simulink model "IEEE34bus_v2019b_Discrete_ZIPload"  (R2019b)
settings: Solver=ode4  StartTime=0.0  StopTime=5  FixedStep=Ts  MaxStep=1e-4  RelTol=1e-4
InitFcn:
  | a=1; % Loading Factor
  | Ts=50e-6;
  | % phase to sequence conversion of RXB matrices
  | c=1*exp(sqrt(-1)*(120*pi/180));
  | T=[1 1 1;1 c*c c;1 c c*c];
  | Tinv=1/3*[1 1 1;1 c c*c;1 c*c c];
  | 
  | % Simulation data for the IEEE 34 Node Test Feeder model
  | mi2km = 1.60934;%  miles to km conversion
  | ft2km = 0.0003048; % feet to km conversion
  | ms2F = 1*1e-6/(2*pi*60);% microsiemens to Farads conversion
  | 
  | %% Configuration 300 - series reactance - ohm/mile
  | R_300 = [1.3368 0.2101 0.2130;0.2101 1.3238 0.2066;0.2130 0.2066 1.3294];
  | X_300 = [1.3343 0.5779 0.5015;0.5779 1.3569 0.4591;0.5015 0.4591 1.3471];
  | % charging susceptance - microsiemens/mile
  | B_300 = [5.3350 -1.5313 -0.9943;-1.5313 5.0979 -0.6212;-0.9943 -0.6212 4.8880];
  | 
  | R_300 = R_300/mi2km;
  | Rseq=Tinv*R_300*T;
  | R1_300=Rseq(2,2);R0_300=Rseq(1,1);
  | 
  | L_300 = (X_300/(2*pi*60))/mi2km;
  | Lseq=Tinv*L_300*T;
  | L1_300=Lseq(2,2);L0_300=Lseq(1,1);
  | 
  | C_300 =(B_300*ms2F)/mi2km;
  | Cseq=Tinv*C_300*T;
  | C1_300=Cseq(2,2);C0_300=Cseq(1,1);
  | 
  | %% Configuration 301 - series reactance - ohm/mile
  | R_301 = [1.9300 0.2327 0.2359;0.2327 1.9157 0.2288;0.2359 0.2288 1.9219];
  | X_301 = [1.4115 0.6442 0.5691;0.6442 1.4281 0.5238;0.5691 0.5238 1.4209];
  | % charging susceptance - microsiemens/mile
  | B_301 = [5.1207 -1.4364 -0.9402;-1.4364 4.9055 -0.5951;-0.9402 -0.5951 4.7154];
  | 
  | R_301 = R_301/mi2km;
  | Rseq=Tinv*R_301*T;
  | R1_301=Rseq(2,2);R0_301=Rseq(1,1);
  | 
  | L_301 = (X_301/(2*pi*60))/mi2km;
  | Lseq=Tinv*L_301*T;
  | L1_301=Lseq(2,2);L0_301=Lseq(1,1);
  | 
  | C_301 =(B_301*ms2F)/mi2km;
  | Cseq=Tinv*C_301*T;
  | C1_301=Cseq(2,2);C0_301=Cseq(1,1);
  | 
  | %% Configuration 302 - series reactance - ohm/mile
  | R_302 = [2.7995 0 0;0 0 0;0 0 0];
  | X_302 = [1.4855 0 0;0 0 0;0 0 0];
  | % charging susceptance - microsiemens/mile
  | B_302 = [4.2251 0 0;0 0 0;0 0 0];
  | 
  | R_302 = R_302/mi2km;
  | Rseq=Tinv*R_302*T;
  | R1_302=Rseq(2,2);R0_302=Rseq(1,1);
  | 
  | L_302 = (X_302/(2*pi*60))/mi2km;
  | Lseq=Tinv*L_302*T;
  | ... (+41 lines)
undefined symbols (not defined in the file): find_system
libraries: powerlib x552, powerlib_meascontrol x162
(part 9 of 9)

== matlab function IEEE34bus_v2019b_Discrete_ZIPload/860 D PQ/Embedded MATLAB Function1 ==
  data: Iinjinst output; Vmeas input; LoadType parameter; Vnom parameter; Pnom parameter; Qnom parameter; Vlim parameter; fnom parameter; clock input; Ddel input
%Three Phase Delta ZIP Load
%Author: Arun Suresh, University of North Carolina, Charlotte
%Pl=Pnom(Kz*(Vmeas/Vnom)^2+Ki(Vmeas/Vnom)+Kp), nom-nominal value,meas-measured value
%Ql=Qnom(Kz*(Vmeas/Vnom)^2+Ki(Vmeas/Vnom)+Kp), nom-nominal value,meas-measured value
%Iinj=((Pl+jQl)/Vmeas)'
function Iinjinst  = InjectedCurrent(Vmeas,LoadType,Vnom,Pnom,Qnom,Vlim,fnom,clock,Ddel)
% Calculate Pl and Ql.
Kz=0;Ki=0;Kp=0;
Vk=abs(Vmeas/(Vnom));%(Vmeas/Vnom)
switch LoadType  % 1 for Constant Z, 2 for Constant I and 3 for Constant P, 
    case 1
        Kz=1;
    case 2
        if Vk >= Vlim % convert to Constant Z load due to voltage violation
            Ki=1;
        else
            Kz=1;
        end
    case 3
        if Vk >= Vlim % convert to Constant Z load due to voltage violation
           Kp=1;
        else
            Kz=1;
        end          
 
end
Pl=Pnom'.*((Kz*Vk.*Vk)+(Ki*Vk)+(Kp));
Ql=Qnom'.*((Kz*Vk.*Vk)+(Ki*Vk)+(Kp));
% Net Injected Curent.
% j=sqrt(-1);
Iinj = conj((Pl+j*Ql)./Vmeas);
Iinjinsta =abs(Iinj(1))*sqrt(2)*sin(2*fnom*pi*clock + angle(Iinj(1))+Ddel(1));
Iinjinstb =abs(Iinj(2))*sqrt(2)*sin(2*fnom*pi*clock + angle(Iinj(2))+Ddel(2));
Iinjinstc =abs(Iinj(3))*sqrt(2)*sin(2*fnom*pi*clock + angle(Iinj(3))+Ddel(3));
Iinjinst=[Iinjinsta  Iinjinstb  Iinjinstc]';

== matlab function IEEE34bus_v2019b_Discrete_ZIPload/860 Y PQ/Embedded MATLAB Function1 ==
  data: Iinjinst output; Vmeas input; LoadType parameter; Vnom parameter; Pnom parameter; Qnom parameter; Vlim parameter; fnom parameter; clock input; Ddel input
%Three Phase Star ZIP Load
%Author: Arun Suresh, University of North Carolina, Charlotte
%Pl=Pnom(Kz*(Vmeas/Vnom)^2+Ki(Vmeas/Vnom)+Kp), nom-nominal value,meas-measured value
%Ql=Qnom(Kz*(Vmeas/Vnom)^2+Ki(Vmeas/Vnom)+Kp), nom-nominal value,meas-measured value
%Iinj=((Pl+jQl)/Vmeas)'
function Iinjinst  = InjectedCurrent(Vmeas,LoadType,Vnom,Pnom,Qnom,Vlim,fnom,clock,Ddel)
% Calculate Pl and Ql.
Kz=0;Ki=0;Kp=0;
Vk=abs(Vmeas/(Vnom/sqrt(3)));%(Vmeas/Vnom)
switch LoadType  % 1 for Constant Z, 2 for Constant I and 3 for Constant P, 
    case 1
        Kz=1;
    case 2
        if Vk >= Vlim % convert to Constant Z load due to voltage violation
            Ki=1;
        else
            Kz=1;
        end
    case 3
        if Vk >= Vlim % convert to Constant Z load due to voltage violation
           Kp=1;
        else
            Kz=1;
        end          
 
end
Pl=Pnom'.*((Kz*Vk.*Vk)+(Ki*Vk)+(Kp));
Ql=Qnom'.*((Kz*Vk.*Vk)+(Ki*Vk)+(Kp));
% Net Injected Curent.
% j=sqrt(-1);
Iinj = conj((Pl+j*Ql)./Vmeas);
Iinjinsta =abs(Iinj(1))*sqrt(2)*sin(2*fnom*pi*clock + angle(Iinj(1))+Ddel(1));
Iinjinstb =abs(Iinj(2))*sqrt(2)*sin(2*fnom*pi*clock + angle(Iinj(2))+Ddel(2));
Iinjinstc =abs(Iinj(3))*sqrt(2)*sin(2*fnom*pi*clock + angle(Iinj(3))+Ddel(3));
Iinjinst=[Iinjinsta  Iinjinstb  Iinjinstc]';

== matlab function IEEE34bus_v2019b_Discrete_ZIPload/836 D PQ/Embedded MATLAB Function1 ==
  data: Iinjinst output; Vmeas input; LoadType parameter; Vnom parameter; Pnom parameter; Qnom parameter; Vlim parameter; fnom parameter; clock input; Ddel input
%Three Phase Delta ZIP Load
%Author: Arun Suresh, University of North Carolina, Charlotte
%Pl=Pnom(Kz*(Vmeas/Vnom)^2+Ki(Vmeas/Vnom)+Kp), nom-nominal value,meas-measured value
%Ql=Qnom(Kz*(Vmeas/Vnom)^2+Ki(Vmeas/Vnom)+Kp), nom-nominal value,meas-measured value
%Iinj=((Pl+jQl)/Vmeas)'
function Iinjinst  = InjectedCurrent(Vmeas,LoadType,Vnom,Pnom,Qnom,Vlim,fnom,clock,Ddel)
% Calculate Pl and Ql.
Kz=0;Ki=0;Kp=0;
Vk=abs(Vmeas/(Vnom));%(Vmeas/Vnom)
switch LoadType  % 1 for Constant Z, 2 for Constant I and 3 for Constant P, 
    case 1
        Kz=1;
    case 2
        if Vk >= Vlim % convert to Constant Z load due to voltage violation
            Ki=1;
        else
            Kz=1;
        end
    case 3
        if Vk >= Vlim % convert to Constant Z load due to voltage violation
           Kp=1;
        else
            Kz=1;
        end          
 
end
Pl=Pnom'.*((Kz*Vk.*Vk)+(Ki*Vk)+(Kp));
Ql=Qnom'.*((Kz*Vk.*Vk)+(Ki*Vk)+(Kp));
% Net Injected Curent.
% j=sqrt(-1);
Iinj = conj((Pl+j*Ql)./Vmeas);
Iinjinsta =abs(Iinj(1))*sqrt(2)*sin(2*fnom*pi*clock + angle(Iinj(1))+Ddel(1));
Iinjinstb =abs(Iinj(2))*sqrt(2)*sin(2*fnom*pi*clock + angle(Iinj(2))+Ddel(2));
Iinjinstc =abs(Iinj(3))*sqrt(2)*sin(2*fnom*pi*clock + angle(Iinj(3))+Ddel(3));
Iinjinst=[Iinjinsta  Iinjinstb  Iinjinstc]';

== matlab function IEEE34bus_v2019b_Discrete_ZIPload/836 D I/Embedded MATLAB Function1 ==
  data: Iinjinst output; Vmeas input; LoadType parameter; Vnom parameter; Pnom parameter; Qnom parameter; Vlim parameter; fnom parameter; clock input; Ddel input
%Three Phase Delta ZIP Load
%Author: Arun Suresh, University of North Carolina, Charlotte
%Pl=Pnom(Kz*(Vmeas/Vnom)^2+Ki(Vmeas/Vnom)+Kp), nom-nominal value,meas-measured value
%Ql=Qnom(Kz*(Vmeas/Vnom)^2+Ki(Vmeas/Vnom)+Kp), nom-nominal value,meas-measured value
%Iinj=((Pl+jQl)/Vmeas)'
function Iinjinst  = InjectedCurrent(Vmeas,LoadType,Vnom,Pnom,Qnom,Vlim,fnom,clock,Ddel)
% Calculate Pl and Ql.
Kz=0;Ki=0;Kp=0;
Vk=abs(Vmeas/(Vnom));%(Vmeas/Vnom)
switch LoadType  % 1 for Constant Z, 2 for Constant I and 3 for Constant P, 
    case 1
        Kz=1;
    case 2
        if Vk >= Vlim % convert to Constant Z load due to voltage violation
            Ki=1;
        else
            Kz=1;
        end
    case 3
        if Vk >= Vlim % convert to Constant Z load due to voltage violation
           Kp=1;
        else
            Kz=1;
        end          
 
end
Pl=Pnom'.*((Kz*Vk.*Vk)+(Ki*Vk)+(Kp));
Ql=Qnom'.*((Kz*Vk.*Vk)+(Ki*Vk)+(Kp));
% Net Injected Curent.
% j=sqrt(-1);
Iinj = conj((Pl+j*Ql)./Vmeas);
Iinjinsta =abs(Iinj(1))*sqrt(2)*sin(2*fnom*pi*clock + angle(Iinj(1))+Ddel(1));
Iinjinstb =abs(Iinj(2))*sqrt(2)*sin(2*fnom*pi*clock + angle(Iinj(2))+Ddel(2));
Iinjinstc =abs(Iinj(3))*sqrt(2)*sin(2*fnom*pi*clock + angle(Iinj(3))+Ddel(3));
Iinjinst=[Iinjinsta  Iinjinstb  Iinjinstc]';

== matlab function IEEE34bus_v2019b_Discrete_ZIPload/840 D I/Embedded MATLAB Function1 ==
  data: Iinjinst output; Vmeas input; LoadType parameter; Vnom parameter; Pnom parameter; Qnom parameter; Vlim parameter; fnom parameter; clock input; Ddel input
%Three Phase Delta ZIP Load
%Author: Arun Suresh, University of North Carolina, Charlotte
%Pl=Pnom(Kz*(Vmeas/Vnom)^2+Ki(Vmeas/Vnom)+Kp), nom-nominal value,meas-measured value
%Ql=Qnom(Kz*(Vmeas/Vnom)^2+Ki(Vmeas/Vnom)+Kp), nom-nominal value,meas-measured value
%Iinj=((Pl+jQl)/Vmeas)'
function Iinjinst  = InjectedCurrent(Vmeas,LoadType,Vnom,Pnom,Qnom,Vlim,fnom,clock,Ddel)
% Calculate Pl and Ql.
Kz=0;Ki=0;Kp=0;
Vk=abs(Vmeas/(Vnom));%(Vmeas/Vnom)
switch LoadType  % 1 for Constant Z, 2 for Constant I and 3 for Constant P, 
    case 1
        Kz=1;
    case 2
        if Vk >= Vlim % convert to Constant Z load due to voltage violation
            Ki=1;
        else
            Kz=1;
        end
    case 3
        if Vk >= Vlim % convert to Constant Z load due to voltage violation
           Kp=1;
        else
            Kz=1;
        end          
 
end
Pl=Pnom'.*((Kz*Vk.*Vk)+(Ki*Vk)+(Kp));
Ql=Qnom'.*((Kz*Vk.*Vk)+(Ki*Vk)+(Kp));
% Net Injected Curent.
% j=sqrt(-1);
Iinj = conj((Pl+j*Ql)./Vmeas);
Iinjinsta =abs(Iinj(1))*sqrt(2)*sin(2*fnom*pi*clock + angle(Iinj(1))+Ddel(1));
Iinjinstb =abs(Iinj(2))*sqrt(2)*sin(2*fnom*pi*clock + angle(Iinj(2))+Ddel(2));
Iinjinstc =abs(Iinj(3))*sqrt(2)*sin(2*fnom*pi*clock + angle(Iinj(3))+Ddel(3));
Iinjinst=[Iinjinsta  Iinjinstb  Iinjinstc]';

== matlab function IEEE34bus_v2019b_Discrete_ZIPload/840 Y I/Embedded MATLAB Function1 ==
  data: Iinjinst output; Vmeas input; LoadType parameter; Vnom parameter; Pnom parameter; Qnom parameter; Vlim parameter; fnom parameter; clock input; Ddel input
%Three Phase Star ZIP Load
%Author: Arun Suresh, University of North Carolina, Charlotte
%Pl=Pnom(Kz*(Vmeas/Vnom)^2+Ki(Vmeas/Vnom)+Kp), nom-nominal value,meas-measured value
%Ql=Qnom(Kz*(Vmeas/Vnom)^2+Ki(Vmeas/Vnom)+Kp), nom-nominal value,meas-measured value
%Iinj=((Pl+jQl)/Vmeas)'
function Iinjinst  = InjectedCurrent(Vmeas,LoadType,Vnom,Pnom,Qnom,Vlim,fnom,clock,Ddel)
% Calculate Pl and Ql.
Kz=0;Ki=0;Kp=0;
Vk=abs(Vmeas/(Vnom/sqrt(3)));%(Vmeas/Vnom)
switch LoadType  % 1 for Constant Z, 2 for Constant I and 3 for Constant P, 
    case 1
        Kz=1;
    case 2
        if Vk >= Vlim % convert to Constant Z load due to voltage violation
            Ki=1;
        else
            Kz=1;
        end
    case 3
        if Vk >= Vlim % convert to Constant Z load due to voltage violation
           Kp=1;
        else
            Kz=1;
        end          
 
end
Pl=Pnom'.*((Kz*Vk.*Vk)+(Ki*Vk)+(Kp));
Ql=Qnom'.*((Kz*Vk.*Vk)+(Ki*Vk)+(Kp));
% Net Injected Curent.
% j=sqrt(-1);
Iinj = conj((Pl+j*Ql)./Vmeas);
Iinjinsta =abs(Iinj(1))*sqrt(2)*sin(2*fnom*pi*clock + angle(Iinj(1))+Ddel(1));
Iinjinstb =abs(Iinj(2))*sqrt(2)*sin(2*fnom*pi*clock + angle(Iinj(2))+Ddel(2));
Iinjinstc =abs(Iinj(3))*sqrt(2)*sin(2*fnom*pi*clock + angle(Iinj(3))+Ddel(3));
Iinjinst=[Iinjinsta  Iinjinstb  Iinjinstc]';

== matlab function IEEE34bus_v2019b_Discrete_ZIPload/844 Y PQ/Embedded MATLAB Function ==
  data: Iinjinst output; Vmeas input; LoadType parameter; Vnom parameter; Pnom parameter; Qnom parameter; Vlim parameter; fnom parameter; clock input; Ddel input
%Single Phase ZIP Load
%Author: Arun Suresh, University of North Carolina, Charlotte
%Iinj=((Pnom+jQnom)/Vmeas)'
function Iinjinst = InjectedCurrent(Vmeas,LoadType,Vnom,Pnom,Qnom,Vlim,fnom,clock,Ddel)
% Calculate Pl and Ql.
%  Vmeas=1.2303e+03 + 1.9328e+03i;
Kz=0;Ki=0;Kp=0;
Vk=(abs(Vmeas)/Vnom);%(Vmeas/Vnom)
switch LoadType  % 1 for Constant Z, 2 for Constant I and 3 for Constant P, 
    case 1
        Kz=1;
    case 2
        if Vk >= Vlim % convert to Constant Z load due to voltage violation
            Ki=1;
        else
            Kz=1;
        end
    case 3
        if Vk >= Vlim % convert to Constant Z load due to voltage violation
           Kp=1;
        else
            Kz=1;
        end          
 
end
Pl=Pnom *((Kz*Vk*Vk)+(Ki*Vk)+(Kp));
Ql=Qnom *((Kz*Vk*Vk)+(Ki*Vk)+(Kp));
% Net Injected Curent.
% j=sqrt(-1);
Iinj = conj((Pl+j*Ql)/Vmeas);
Iinjinst =abs(Iinj)*sqrt(2)*sin(2*fnom*pi*clock + angle(Iinj)+Ddel);
yt=Iinj;

== matlab function IEEE34bus_v2019b_Discrete_ZIPload/842 Y PQ/Embedded MATLAB Function ==
  data: Iinjinst output; Vmeas input; LoadType parameter; Vnom parameter; Pnom parameter; Qnom parameter; Vlim parameter; fnom parameter; clock input; Ddel input
%Single Phase ZIP Load
%Author: Arun Suresh, University of North Carolina, Charlotte
%Iinj=((Pnom+jQnom)/Vmeas)'
function Iinjinst = InjectedCurrent(Vmeas,LoadType,Vnom,Pnom,Qnom,Vlim,fnom,clock,Ddel)
% Calculate Pl and Ql.
%  Vmeas=1.2303e+03 + 1.9328e+03i;
Kz=0;Ki=0;Kp=0;
Vk=(abs(Vmeas)/Vnom);%(Vmeas/Vnom)
switch LoadType  % 1 for Constant Z, 2 for Constant I and 3 for Constant P, 
    case 1
        Kz=1;
    case 2
        if Vk >= Vlim % convert to Constant Z load due to voltage violation
            Ki=1;
        else
            Kz=1;
        end
    case 3
        if Vk >= Vlim % convert to Constant Z load due to voltage violation
           Kp=1;
        else
            Kz=1;
        end          
 
end
Pl=Pnom *((Kz*Vk*Vk)+(Ki*Vk)+(Kp));
Ql=Qnom *((Kz*Vk*Vk)+(Ki*Vk)+(Kp));
% Net Injected Curent.
% j=sqrt(-1);
Iinj = conj((Pl+j*Ql)/Vmeas);
Iinjinst =abs(Iinj)*sqrt(2)*sin(2*fnom*pi*clock + angle(Iinj)+Ddel);
yt=Iinj;

== matlab function IEEE34bus_v2019b_Discrete_ZIPload/844 Y Z/Embedded MATLAB Function1 ==
  data: Iinjinst output; Vmeas input; LoadType parameter; Vnom parameter; Pnom parameter; Qnom parameter; Vlim parameter; fnom parameter; clock input; Ddel input
%Three Phase Star ZIP Load
%Author: Arun Suresh, University of North Carolina, Charlotte
%Pl=Pnom(Kz*(Vmeas/Vnom)^2+Ki(Vmeas/Vnom)+Kp), nom-nominal value,meas-measured value
%Ql=Qnom(Kz*(Vmeas/Vnom)^2+Ki(Vmeas/Vnom)+Kp), nom-nominal value,meas-measured value
%Iinj=((Pl+jQl)/Vmeas)'
function Iinjinst  = InjectedCurrent(Vmeas,LoadType,Vnom,Pnom,Qnom,Vlim,fnom,clock,Ddel)
% Calculate Pl and Ql.
Kz=0;Ki=0;Kp=0;
Vk=abs(Vmeas/(Vnom/sqrt(3)));%(Vmeas/Vnom)
switch LoadType  % 1 for Constant Z, 2 for Constant I and 3 for Constant P, 
    case 1
        Kz=1;
    case 2
        if Vk >= Vlim % convert to Constant Z load due to voltage violation
            Ki=1;
        else
            Kz=1;
        end
    case 3
        if Vk >= Vlim % convert to Constant Z load due to voltage violation
           Kp=1;
        else
            Kz=1;
        end          
 
end
Pl=Pnom'.*((Kz*Vk.*Vk)+(Ki*Vk)+(Kp));
Ql=Qnom'.*((Kz*Vk.*Vk)+(Ki*Vk)+(Kp));
% Net Injected Curent.
% j=sqrt(-1);
Iinj = conj((Pl+j*Ql)./Vmeas);
Iinjinsta =abs(Iinj(1))*sqrt(2)*sin(2*fnom*pi*clock + angle(Iinj(1))+Ddel(1));
Iinjinstb =abs(Iinj(2))*sqrt(2)*sin(2*fnom*pi*clock + angle(Iinj(2))+Ddel(2));
Iinjinstc =abs(Iinj(3))*sqrt(2)*sin(2*fnom*pi*clock + angle(Iinj(3))+Ddel(3));
Iinjinst=[Iinjinsta  Iinjinstb  Iinjinstc]';

== matlab function IEEE34bus_v2019b_Discrete_ZIPload/846 Y PQ/Embedded MATLAB Function1 ==
  data: Iinjinst output; Vmeas input; LoadType parameter; Vnom parameter; Pnom parameter; Qnom parameter; Vlim parameter; fnom parameter; clock input; Ddel input
%Three Phase Star ZIP Load
%Author: Arun Suresh, University of North Carolina, Charlotte
%Pl=Pnom(Kz*(Vmeas/Vnom)^2+Ki(Vmeas/Vnom)+Kp), nom-nominal value,meas-measured value
%Ql=Qnom(Kz*(Vmeas/Vnom)^2+Ki(Vmeas/Vnom)+Kp), nom-nominal value,meas-measured value
%Iinj=((Pl+jQl)/Vmeas)'
function Iinjinst  = InjectedCurrent(Vmeas,LoadType,Vnom,Pnom,Qnom,Vlim,fnom,clock,Ddel)
% Calculate Pl and Ql.
Kz=0;Ki=0;Kp=0;
Vk=abs(Vmeas/(Vnom/sqrt(3)));%(Vmeas/Vnom)
switch LoadType  % 1 for Constant Z, 2 for Constant I and 3 for Constant P, 
    case 1
        Kz=1;
    case 2
        if Vk >= Vlim % convert to Constant Z load due to voltage violation
            Ki=1;
        else
            Kz=1;
        end
    case 3
        if Vk >= Vlim % convert to Constant Z load due to voltage violation
           Kp=1;
        else
            Kz=1;
        end          
 
end
Pl=Pnom'.*((Kz*Vk.*Vk)+(Ki*Vk)+(Kp));
Ql=Qnom'.*((Kz*Vk.*Vk)+(Ki*Vk)+(Kp));
% Net Injected Curent.
% j=sqrt(-1);
Iinj = conj((Pl+j*Ql)./Vmeas);
Iinjinsta =abs(Iinj(1))*sqrt(2)*sin(2*fnom*pi*clock + angle(Iinj(1))+Ddel(1));
Iinjinstb =abs(Iinj(2))*sqrt(2)*sin(2*fnom*pi*clock + angle(Iinj(2))+Ddel(2));
Iinjinstc =abs(Iinj(3))*sqrt(2)*sin(2*fnom*pi*clock + angle(Iinj(3))+Ddel(3));
Iinjinst=[Iinjinsta  Iinjinstb  Iinjinstc]';

== matlab function IEEE34bus_v2019b_Discrete_ZIPload/844 Y PQ1/Embedded MATLAB Function1 ==
  data: Iinjinst output; Vmeas input; LoadType parameter; Vnom parameter; Pnom parameter; Qnom parameter; Vlim parameter; fnom parameter; clock input; Ddel input
%Three Phase Star ZIP Load
%Author: Arun Suresh, University of North Carolina, Charlotte
%Pl=Pnom(Kz*(Vmeas/Vnom)^2+Ki(Vmeas/Vnom)+Kp), nom-nominal value,meas-measured value
%Ql=Qnom(Kz*(Vmeas/Vnom)^2+Ki(Vmeas/Vnom)+Kp), nom-nominal value,meas-measured value
%Iinj=((Pl+jQl)/Vmeas)'
function Iinjinst  = InjectedCurrent(Vmeas,LoadType,Vnom,Pnom,Qnom,Vlim,fnom,clock,Ddel)
% Calculate Pl and Ql.
Kz=0;Ki=0;Kp=0;
Vk=abs(Vmeas/(Vnom/sqrt(3)));%(Vmeas/Vnom)
switch LoadType  % 1 for Constant Z, 2 for Constant I and 3 for Constant P, 
    case 1
        Kz=1;
    case 2
        if Vk >= Vlim % convert to Constant Z load due to voltage violation
            Ki=1;
        else
            Kz=1;
        end
    case 3
        if Vk >= Vlim % convert to Constant Z load due to voltage violation
           Kp=1;
        else
            Kz=1;
        end          
 
end
Pl=Pnom'.*((Kz*Vk.*Vk)+(Ki*Vk)+(Kp));
Ql=Qnom'.*((Kz*Vk.*Vk)+(Ki*Vk)+(Kp));
% Net Injected Curent.
% j=sqrt(-1);
Iinj = conj((Pl+j*Ql)./Vmeas);
Iinjinsta =abs(Iinj(1))*sqrt(2)*sin(2*fnom*pi*clock + angle(Iinj(1))+Ddel(1));
Iinjinstb =abs(Iinj(2))*sqrt(2)*sin(2*fnom*pi*clock + angle(Iinj(2))+Ddel(2));
Iinjinstc =abs(Iinj(3))*sqrt(2)*sin(2*fnom*pi*clock + angle(Iinj(3))+Ddel(3));
Iinjinst=[Iinjinsta  Iinjinstb  Iinjinstc]';

== matlab function IEEE34bus_v2019b_Discrete_ZIPload/848 Y PQ/Embedded MATLAB Function ==
  data: Iinjinst output; Vmeas input; LoadType parameter; Vnom parameter; Pnom parameter; Qnom parameter; Vlim parameter; fnom parameter; clock input; Ddel input
%Single Phase ZIP Load
%Author: Arun Suresh, University of North Carolina, Charlotte
%Iinj=((Pnom+jQnom)/Vmeas)'
function Iinjinst = InjectedCurrent(Vmeas,LoadType,Vnom,Pnom,Qnom,Vlim,fnom,clock,Ddel)
% Calculate Pl and Ql.
%  Vmeas=1.2303e+03 + 1.9328e+03i;
Kz=0;Ki=0;Kp=0;
Vk=(abs(Vmeas)/Vnom);%(Vmeas/Vnom)
switch LoadType  % 1 for Constant Z, 2 for Constant I and 3 for Constant P, 
    case 1
        Kz=1;
    case 2
        if Vk >= Vlim % convert to Constant Z load due to voltage violation
            Ki=1;
        else
            Kz=1;
        end
    case 3
        if Vk >= Vlim % convert to Constant Z load due to voltage violation
           Kp=1;
        else
            Kz=1;
        end          
 
end
Pl=Pnom *((Kz*Vk*Vk)+(Ki*Vk)+(Kp));
Ql=Qnom *((Kz*Vk*Vk)+(Ki*Vk)+(Kp));
% Net Injected Curent.
% j=sqrt(-1);
Iinj = conj((Pl+j*Ql)/Vmeas);
Iinjinst =abs(Iinj)*sqrt(2)*sin(2*fnom*pi*clock + angle(Iinj)+Ddel);
yt=Iinj;

== matlab function IEEE34bus_v2019b_Discrete_ZIPload/846 Y PQ1/Embedded MATLAB Function ==
  data: Iinjinst output; Vmeas input; LoadType parameter; Vnom parameter; Pnom parameter; Qnom parameter; Vlim parameter; fnom parameter; clock input; Ddel input
%Single Phase ZIP Load
%Author: Arun Suresh, University of North Carolina, Charlotte
%Iinj=((Pnom+jQnom)/Vmeas)'
function Iinjinst = InjectedCurrent(Vmeas,LoadType,Vnom,Pnom,Qnom,Vlim,fnom,clock,Ddel)
% Calculate Pl and Ql.
%  Vmeas=1.2303e+03 + 1.9328e+03i;
Kz=0;Ki=0;Kp=0;
Vk=(abs(Vmeas)/Vnom);%(Vmeas/Vnom)
switch LoadType  % 1 for Constant Z, 2 for Constant I and 3 for Constant P, 
    case 1
        Kz=1;
    case 2
        if Vk >= Vlim % convert to Constant Z load due to voltage violation
            Ki=1;
        else
            Kz=1;
        end
    case 3
        if Vk >= Vlim % convert to Constant Z load due to voltage violation
           Kp=1;
        else
            Kz=1;
        end          
 
end
Pl=Pnom *((Kz*Vk*Vk)+(Ki*Vk)+(Kp));
Ql=Qnom *((Kz*Vk*Vk)+(Ki*Vk)+(Kp));
% Net Injected Curent.
% j=sqrt(-1);
Iinj = conj((Pl+j*Ql)/Vmeas);
Iinjinst =abs(Iinj)*sqrt(2)*sin(2*fnom*pi*clock + angle(Iinj)+Ddel);
yt=Iinj;

== matlab function IEEE34bus_v2019b_Discrete_ZIPload/848 D PQ/Embedded MATLAB Function1 ==
  data: Iinjinst output; Vmeas input; LoadType parameter; Vnom parameter; Pnom parameter; Qnom parameter; Vlim parameter; fnom parameter; clock input; Ddel input
%Three Phase Delta ZIP Load
%Author: Arun Suresh, University of North Carolina, Charlotte
%Pl=Pnom(Kz*(Vmeas/Vnom)^2+Ki(Vmeas/Vnom)+Kp), nom-nominal value,meas-measured value
%Ql=Qnom(Kz*(Vmeas/Vnom)^2+Ki(Vmeas/Vnom)+Kp), nom-nominal value,meas-measured value
%Iinj=((Pl+jQl)/Vmeas)'
function Iinjinst  = InjectedCurrent(Vmeas,LoadType,Vnom,Pnom,Qnom,Vlim,fnom,clock,Ddel)
% Calculate Pl and Ql.
Kz=0;Ki=0;Kp=0;
Vk=abs(Vmeas/(Vnom));%(Vmeas/Vnom)
switch LoadType  % 1 for Constant Z, 2 for Constant I and 3 for Constant P, 
    case 1
        Kz=1;
    case 2
        if Vk >= Vlim % convert to Constant Z load due to voltage violation
            Ki=1;
        else
            Kz=1;
        end
    case 3
        if Vk >= Vlim % convert to Constant Z load due to voltage violation
           Kp=1;
        else
            Kz=1;
        end          
 
end
Pl=Pnom'.*((Kz*Vk.*Vk)+(Ki*Vk)+(Kp));
Ql=Qnom'.*((Kz*Vk.*Vk)+(Ki*Vk)+(Kp));
% Net Injected Curent.
% j=sqrt(-1);
Iinj = conj((Pl+j*Ql)./Vmeas);
Iinjinsta =abs(Iinj(1))*sqrt(2)*sin(2*fnom*pi*clock + angle(Iinj(1))+Ddel(1));
Iinjinstb =abs(Iinj(2))*sqrt(2)*sin(2*fnom*pi*clock + angle(Iinj(2))+Ddel(2));
Iinjinstc =abs(Iinj(3))*sqrt(2)*sin(2*fnom*pi*clock + angle(Iinj(3))+Ddel(3));
Iinjinst=[Iinjinsta  Iinjinstb  Iinjinstc]';

== matlab function IEEE34bus_v2019b_Discrete_ZIPload/862 Y PQ/Embedded MATLAB Function ==
  data: Iinjinst output; Vmeas input; LoadType parameter; Vnom parameter; Pnom parameter; Qnom parameter; Vlim parameter; fnom parameter; clock input; Ddel input
%Single Phase ZIP Load
%Author: Arun Suresh, University of North Carolina, Charlotte
%Iinj=((Pnom+jQnom)/Vmeas)'
function Iinjinst = InjectedCurrent(Vmeas,LoadType,Vnom,Pnom,Qnom,Vlim,fnom,clock,Ddel)
% Calculate Pl and Ql.
%  Vmeas=1.2303e+03 + 1.9328e+03i;
Kz=0;Ki=0;Kp=0;
Vk=(abs(Vmeas)/Vnom);%(Vmeas/Vnom)
switch LoadType  % 1 for Constant Z, 2 for Constant I and 3 for Constant P, 
    case 1
        Kz=1;
    case 2
        if Vk >= Vlim % convert to Constant Z load due to voltage violation
            Ki=1;
        else
            Kz=1;
        end
    case 3
        if Vk >= Vlim % convert to Constant Z load due to voltage violation
           Kp=1;
        else
            Kz=1;
        end          
 
end
Pl=Pnom *((Kz*Vk*Vk)+(Ki*Vk)+(Kp));
Ql=Qnom *((Kz*Vk*Vk)+(Ki*Vk)+(Kp));
% Net Injected Curent.
% j=sqrt(-1);
Iinj = conj((Pl+j*Ql)/Vmeas);
Iinjinst =abs(Iinj)*sqrt(2)*sin(2*fnom*pi*clock + angle(Iinj)+Ddel);
yt=Iinj;

== matlab function IEEE34bus_v2019b_Discrete_ZIPload/838 Y PQ/Embedded MATLAB Function ==
  data: Iinjinst output; Vmeas input; LoadType parameter; Vnom parameter; Pnom parameter; Qnom parameter; Vlim parameter; fnom parameter; clock input; Ddel input
%Single Phase ZIP Load
%Author: Arun Suresh, University of North Carolina, Charlotte
%Iinj=((Pnom+jQnom)/Vmeas)'
function Iinjinst = InjectedCurrent(Vmeas,LoadType,Vnom,Pnom,Qnom,Vlim,fnom,clock,Ddel)
% Calculate Pl and Ql.
%  Vmeas=1.2303e+03 + 1.9328e+03i;
Kz=0;Ki=0;Kp=0;
Vk=(abs(Vmeas)/Vnom);%(Vmeas/Vnom)
switch LoadType  % 1 for Constant Z, 2 for Constant I and 3 for Constant P, 
    case 1
        Kz=1;
    case 2
        if Vk >= Vlim % convert to Constant Z load due to voltage violation
            Ki=1;
        else
            Kz=1;
        end
    case 3
        if Vk >= Vlim % convert to Constant Z load due to voltage violation
           Kp=1;
        else
            Kz=1;
        end          
 
end
Pl=Pnom *((Kz*Vk*Vk)+(Ki*Vk)+(Kp));
Ql=Qnom *((Kz*Vk*Vk)+(Ki*Vk)+(Kp));
% Net Injected Curent.
% j=sqrt(-1);
Iinj = conj((Pl+j*Ql)/Vmeas);
Iinjinst =abs(Iinj)*sqrt(2)*sin(2*fnom*pi*clock + angle(Iinj)+Ddel);
yt=Iinj;

== matlab function IEEE34bus_v2019b_Discrete_ZIPload/864 Y PQ/Embedded MATLAB Function ==
  data: Iinjinst output; Vmeas input; LoadType parameter; Vnom parameter; Pnom parameter; Qnom parameter; Vlim parameter; fnom parameter; clock input; Ddel input
%Single Phase ZIP Load
%Author: Arun Suresh, University of North Carolina, Charlotte
%Iinj=((Pnom+jQnom)/Vmeas)'
function Iinjinst = InjectedCurrent(Vmeas,LoadType,Vnom,Pnom,Qnom,Vlim,fnom,clock,Ddel)
% Calculate Pl and Ql.
%  Vmeas=1.2303e+03 + 1.9328e+03i;
Kz=0;Ki=0;Kp=0;
Vk=(abs(Vmeas)/Vnom);%(Vmeas/Vnom)
switch LoadType  % 1 for Constant Z, 2 for Constant I and 3 for Constant P, 
    case 1
        Kz=1;
    case 2
        if Vk >= Vlim % convert to Constant Z load due to voltage violation
            Ki=1;
        else
            Kz=1;
        end
    case 3
        if Vk >= Vlim % convert to Constant Z load due to voltage violation
           Kp=1;
        else
            Kz=1;
        end          
 
end
Pl=Pnom *((Kz*Vk*Vk)+(Ki*Vk)+(Kp));
Ql=Qnom *((Kz*Vk*Vk)+(Ki*Vk)+(Kp));
% Net Injected Curent.
% j=sqrt(-1);
Iinj = conj((Pl+j*Ql)/Vmeas);
Iinjinst =abs(Iinj)*sqrt(2)*sin(2*fnom*pi*clock + angle(Iinj)+Ddel);
yt=Iinj;

== matlab function IEEE34bus_v2019b_Discrete_ZIPload/858 Y PQ/Embedded MATLAB Function ==
  data: Iinjinst output; Vmeas input; LoadType parameter; Vnom parameter; Pnom parameter; Qnom parameter; Vlim parameter; fnom parameter; clock input; Ddel input
%Single Phase ZIP Load
%Author: Arun Suresh, University of North Carolina, Charlotte
%Iinj=((Pnom+jQnom)/Vmeas)'
function Iinjinst = InjectedCurrent(Vmeas,LoadType,Vnom,Pnom,Qnom,Vlim,fnom,clock,Ddel)
% Calculate Pl and Ql.
%  Vmeas=1.2303e+03 + 1.9328e+03i;
Kz=0;Ki=0;Kp=0;
Vk=(abs(Vmeas)/Vnom);%(Vmeas/Vnom)
switch LoadType  % 1 for Constant Z, 2 for Constant I and 3 for Constant P, 
    case 1
        Kz=1;
    case 2
        if Vk >= Vlim % convert to Constant Z load due to voltage violation
            Ki=1;
        else
            Kz=1;
        end
    case 3
        if Vk >= Vlim % convert to Constant Z load due to voltage violation
           Kp=1;
        else
            Kz=1;
        end          
 
end
Pl=Pnom *((Kz*Vk*Vk)+(Ki*Vk)+(Kp));
Ql=Qnom *((Kz*Vk*Vk)+(Ki*Vk)+(Kp));
% Net Injected Curent.
% j=sqrt(-1);
Iinj = conj((Pl+j*Ql)/Vmeas);
Iinjinst =abs(Iinj)*sqrt(2)*sin(2*fnom*pi*clock + angle(Iinj)+Ddel);
yt=Iinj;

== matlab function IEEE34bus_v2019b_Discrete_ZIPload/854 Y PQ/Embedded MATLAB Function ==
  data: Iinjinst output; Vmeas input; LoadType parameter; Vnom parameter; Pnom parameter; Qnom parameter; Vlim parameter; fnom parameter; clock input; Ddel input
%Single Phase ZIP Load
%Author: Arun Suresh, University of North Carolina, Charlotte
%Iinj=((Pnom+jQnom)/Vmeas)'
function Iinjinst = InjectedCurrent(Vmeas,LoadType,Vnom,Pnom,Qnom,Vlim,fnom,clock,Ddel)
% Calculate Pl and Ql.
%  Vmeas=1.2303e+03 + 1.9328e+03i;
Kz=0;Ki=0;Kp=0;
Vk=(abs(Vmeas)/Vnom);%(Vmeas/Vnom)
switch LoadType  % 1 for Constant Z, 2 for Constant I and 3 for Constant P, 
    case 1
        Kz=1;
    case 2
        if Vk >= Vlim % convert to Constant Z load due to voltage violation
            Ki=1;
        else
            Kz=1;
        end
    case 3
        if Vk >= Vlim % convert to Constant Z load due to voltage violation
           Kp=1;
        else
            Kz=1;
        end          
 
end
Pl=Pnom *((Kz*Vk*Vk)+(Ki*Vk)+(Kp));
Ql=Qnom *((Kz*Vk*Vk)+(Ki*Vk)+(Kp));
% Net Injected Curent.
% j=sqrt(-1);
Iinj = conj((Pl+j*Ql)/Vmeas);
Iinjinst =abs(Iinj)*sqrt(2)*sin(2*fnom*pi*clock + angle(Iinj)+Ddel);
yt=Iinj;

== matlab function IEEE34bus_v2019b_Discrete_ZIPload/856 Y PQ/Embedded MATLAB Function ==
  data: Iinjinst output; Vmeas input; LoadType parameter; Vnom parameter; Pnom parameter; Qnom parameter; Vlim parameter; fnom parameter; clock input; Ddel input
%Single Phase ZIP Load
%Author: Arun Suresh, University of North Carolina, Charlotte
%Iinj=((Pnom+jQnom)/Vmeas)'
function Iinjinst = InjectedCurrent(Vmeas,LoadType,Vnom,Pnom,Qnom,Vlim,fnom,clock,Ddel)
% Calculate Pl and Ql.
%  Vmeas=1.2303e+03 + 1.9328e+03i;
Kz=0;Ki=0;Kp=0;
Vk=(abs(Vmeas)/Vnom);%(Vmeas/Vnom)
switch LoadType  % 1 for Constant Z, 2 for Constant I and 3 for Constant P, 
    case 1
        Kz=1;
    case 2
        if Vk >= Vlim % convert to Constant Z load due to voltage violation
            Ki=1;
        else
            Kz=1;
        end
    case 3
        if Vk >= Vlim % convert to Constant Z load due to voltage violation
           Kp=1;
        else
            Kz=1;
        end          
 
end
Pl=Pnom *((Kz*Vk*Vk)+(Ki*Vk)+(Kp));
Ql=Qnom *((Kz*Vk*Vk)+(Ki*Vk)+(Kp));
% Net Injected Curent.
% j=sqrt(-1);
Iinj = conj((Pl+j*Ql)/Vmeas);
Iinjinst =abs(Iinj)*sqrt(2)*sin(2*fnom*pi*clock + angle(Iinj)+Ddel);
yt=Iinj;

== matlab function IEEE34bus_v2019b_Discrete_ZIPload/824 Y I/Embedded MATLAB Function ==
  data: Iinjinst output; Vmeas input; LoadType parameter; Vnom parameter; Pnom parameter; Qnom parameter; Vlim parameter; fnom parameter; clock input; Ddel input
%Single Phase ZIP Load
%Author: Arun Suresh, University of North Carolina, Charlotte
%Iinj=((Pnom+jQnom)/Vmeas)'
function Iinjinst = InjectedCurrent(Vmeas,LoadType,Vnom,Pnom,Qnom,Vlim,fnom,clock,Ddel)
% Calculate Pl and Ql.
%  Vmeas=1.2303e+03 + 1.9328e+03i;
Kz=0;Ki=0;Kp=0;
Vk=(abs(Vmeas)/Vnom);%(Vmeas/Vnom)
switch LoadType  % 1 for Constant Z, 2 for Constant I and 3 for Constant P, 
    case 1
        Kz=1;
    case 2
        if Vk >= Vlim % convert to Constant Z load due to voltage violation
            Ki=1;
        else
            Kz=1;
        end
    case 3
        if Vk >= Vlim % convert to Constant Z load due to voltage violation
           Kp=1;
        else
            Kz=1;
        end          
 
end
Pl=Pnom *((Kz*Vk*Vk)+(Ki*Vk)+(Kp));
Ql=Qnom *((Kz*Vk*Vk)+(Ki*Vk)+(Kp));
% Net Injected Curent.
% j=sqrt(-1);
Iinj = conj((Pl+j*Ql)/Vmeas);
Iinjinst =abs(Iinj)*sqrt(2)*sin(2*fnom*pi*clock + angle(Iinj)+Ddel);
yt=Iinj;

== matlab function IEEE34bus_v2019b_Discrete_ZIPload/826 Y I/Embedded MATLAB Function ==
  data: Iinjinst output; Vmeas input; LoadType parameter; Vnom parameter; Pnom parameter; Qnom parameter; Vlim parameter; fnom parameter; clock input; Ddel input
%Single Phase ZIP Load
%Author: Arun Suresh, University of North Carolina, Charlotte
%Iinj=((Pnom+jQnom)/Vmeas)'
function Iinjinst = InjectedCurrent(Vmeas,LoadType,Vnom,Pnom,Qnom,Vlim,fnom,clock,Ddel)
% Calculate Pl and Ql.
%  Vmeas=1.2303e+03 + 1.9328e+03i;
Kz=0;Ki=0;Kp=0;
Vk=(abs(Vmeas)/Vnom);%(Vmeas/Vnom)
switch LoadType  % 1 for Constant Z, 2 for Constant I and 3 for Constant P, 
    case 1
        Kz=1;
    case 2
        if Vk >= Vlim % convert to Constant Z load due to voltage violation
            Ki=1;
        else
            Kz=1;
        end
    case 3
        if Vk >= Vlim % convert to Constant Z load due to voltage violation
           Kp=1;
        else
            Kz=1;
        end          
 
end
Pl=Pnom *((Kz*Vk*Vk)+(Ki*Vk)+(Kp));
Ql=Qnom *((Kz*Vk*Vk)+(Ki*Vk)+(Kp));
% Net Injected Curent.
% j=sqrt(-1);
Iinj = conj((Pl+j*Ql)/Vmeas);
Iinjinst =abs(Iinj)*sqrt(2)*sin(2*fnom*pi*clock + angle(Iinj)+Ddel);
yt=Iinj;
